simulink model "reactor_2"  (R2021a)
settings: Solver=VariableStepAuto  StartTime=0.0  StopTime=10.0  RelTol=1e-3
values from neighbouring files (symbols this model uses):
  c0 = 5.4698    [script.m]
  ci = 10    [script.m]
  EdR = 49584/8.32    (= 5959.61538462)    [script.m]
  hA = kT*At    (= 18821.555234)    [script.m]
  k0 = 34930800    [script.m]
  mdH = 24953    [script.m]
  q = 10    [script.m]
  rcp = 2093    [script.m]
  T0 = 339.437    [script.m]
  Ti = 38+273    (= 311)    [script.m]
  Tr = Tri    (= 311)    [script.m]
  V = 10    [script.m]
settings Model: Creator=Automatica  LastModifiedBy=Automatica

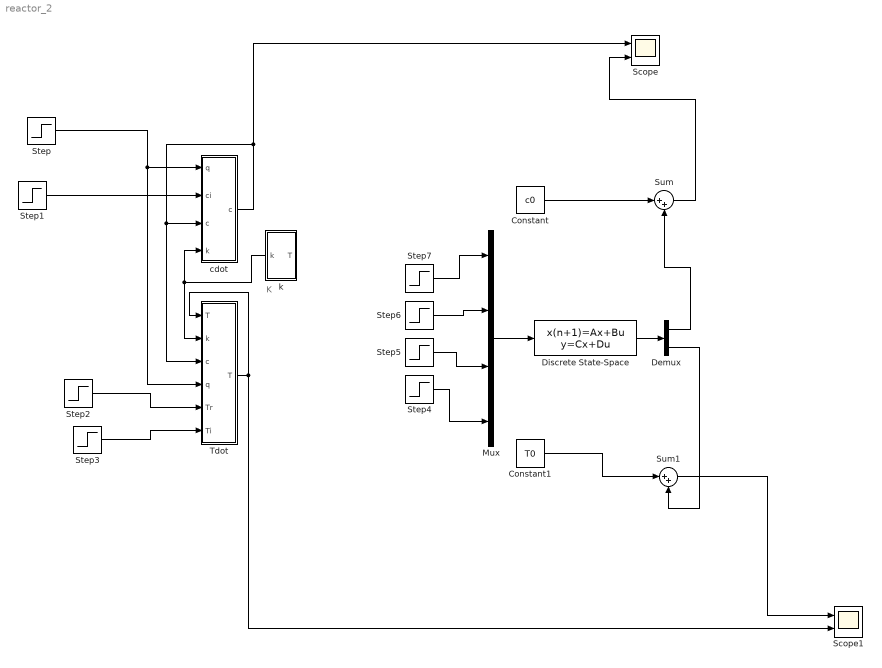
== system reactor_2 ==
  note: K
  Constant : Constant  Value=c0
  Constant1 : Constant  Value=T0
  Demux : Demux  Outputs=2
  Discrete State-Space : DiscreteStateSpace  SampleTime=-1
  Mux : Mux
  Scope : Scope  NumInputPorts=2
  Scope1 : Scope  NumInputPorts=2
  Step : Step  Time=0  Before=q  After=1.1*q  SampleTime=0
  Step1 : Step  Time=0  Before=ci  After=1.1*ci  SampleTime=0
  Step2 : Step  Time=0  Before=Tr  After=1.1*Tr  SampleTime=0
  Step3 : Step  Time=0  Before=Ti  After=1.1*Ti  SampleTime=0
  Step4 : Step  Time=0  After=0.1*Ti  SampleTime=0
  Step5 : Step  Time=0  After=0.1*Tr  SampleTime=0
  Step6 : Step  Time=0  After=0.1*ci  SampleTime=0
  Step7 : Step  Time=0  After=0.1*q  SampleTime=0
  Sum : Sum  Inputs=|++
  Sum1 : Sum  Inputs=|++
  Tdot : Subsystem
  cdot : Subsystem
  k : Subsystem
  wires:
  Step2/1 -> Tdot/5(Tr)
  Step1/1 -> cdot/2(ci)
  Step3/1 -> Tdot/6(Ti)
  Step/1 -> cdot/1(q), Tdot/4(q)
  Tdot/1("T  ") -> Scope1/2, Tdot/1(T)
  cdot/1(c) -> Scope/1, cdot/3("c  "), Tdot/3(c)
  Step7/1 -> Mux/1
  Step6/1 -> Mux/2
  Step5/1 -> Mux/3
  Step4/1 -> Mux/4
  Mux/1 -> Discrete State-Space/1
  Discrete State-Space/1 -> Demux/1
  Demux/1 -> Sum/2
  Constant/1 -> Sum/1
  Sum/1 -> Scope/2
  Constant1/1 -> Sum1/1
  Demux/2 -> Sum1/2
  Sum1/1 -> Scope1/1
  k/1(k) -> Tdot/2(k), cdot/4(k)

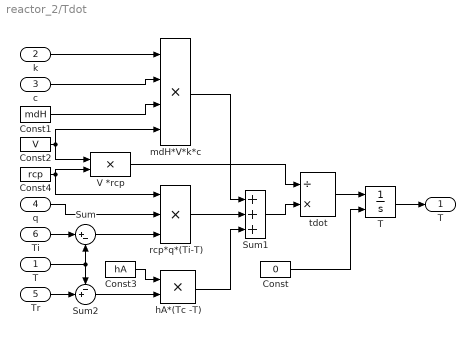
== system reactor_2/Tdot ==
  T : Inport  Interpolate=off
  k : Inport  Port=2  Interpolate=off
  c : Inport  Port=3  Interpolate=off
  q : Inport  Port=4  Interpolate=off
  Tr : Inport  Port=5  Interpolate=off
  Ti : Inport  Port=6  Interpolate=off
  Const : Constant  Value=0
  Const1 : Constant  Value=mdH
  Const2 : Constant  Value=V
  Const3 : Constant  Value=hA
  Const4 : Constant  Value=rcp
  Sum : Sum  Inputs=|+-  InputSameDT=on  SaturateOnIntegerOverflow=on  OutDataTypeStr=Inherit: Same as first input
  Sum1 : Sum  Inputs=+++  InputSameDT=on  SaturateOnIntegerOverflow=on  OutDataTypeStr=Inherit: Same as first input
  Sum2 : Sum  Inputs=-+|  InputSameDT=on  SaturateOnIntegerOverflow=on  OutDataTypeStr=Inherit: Same as first input
  "T " : Integrator  InitialConditionSource=external
  V *rcp : Product  Inputs=**  InputSameDT=on  RndMeth=Zero  SaturateOnIntegerOverflow=on  OutDataTypeStr=Inherit: Same as first input
  hA*(Tc -T) : Product  Inputs=**  InputSameDT=on  RndMeth=Zero  SaturateOnIntegerOverflow=on  OutDataTypeStr=Inherit: Same as first input
  mdH*V*k*c : Product  Inputs=****  InputSameDT=on  RndMeth=Zero  SaturateOnIntegerOverflow=on  OutDataTypeStr=Inherit: Same as first input
  rcp*q*(Ti-T) : Product  Inputs=***  InputSameDT=on  RndMeth=Zero  SaturateOnIntegerOverflow=on  OutDataTypeStr=Inherit: Same as first input
  tdot : Product  Inputs=/*  InputSameDT=on  RndMeth=Zero  SaturateOnIntegerOverflow=on  OutDataTypeStr=Inherit: Same as first input
  "T  " : Outport
  wires:
  Ti/1 -> Sum/1
  Sum/1 -> rcp*q*(Ti-T)/3
  q/1 -> rcp*q*(Ti-T)/2
  T/1 -> Sum/2, Sum2/1
  Tr/1 -> Sum2/2
  Sum2/1 -> hA*(Tc -T)/2
  Const3/1 -> hA*(Tc -T)/1
  k/1 -> mdH*V*k*c/1
  c/1 -> mdH*V*k*c/2
  Const1/1 -> mdH*V*k*c/3
  mdH*V*k*c/1 -> Sum1/1
  rcp*q*(Ti-T)/1 -> Sum1/2
  hA*(Tc -T)/1 -> Sum1/3
  Const2/1 -> mdH*V*k*c/4, V *rcp/1
  Const4/1 -> rcp*q*(Ti-T)/1, V *rcp/2
  V *rcp/1 -> tdot/1
  Sum1/1 -> tdot/2
  tdot/1 -> "T "/1
  Const/1 -> "T "/2
  "T "/1 -> "T  "/1

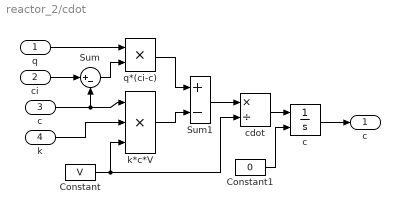
== system reactor_2/cdot ==
  q : Inport  Interpolate=off
  ci : Inport  Port=2  Interpolate=off
  "c  " : Inport  Port=3  Interpolate=off
  k : Inport  Port=4  Interpolate=off
  Constant : Constant  Value=V
  Constant1 : Constant  Value=0
  Sum : Sum  Inputs=|+-  InputSameDT=on  SaturateOnIntegerOverflow=on  OutDataTypeStr=Inherit: Same as first input
  Sum1 : Sum  Inputs=+-  InputSameDT=on  SaturateOnIntegerOverflow=on  OutDataTypeStr=Inherit: Same as first input
  "c " : Integrator  InitialConditionSource=external
  cdot : Product  Inputs=*/  InputSameDT=on  RndMeth=Zero  SaturateOnIntegerOverflow=on  OutDataTypeStr=Inherit: Same as first input
  k*c*V : Product  Inputs=***  InputSameDT=on  RndMeth=Zero  SaturateOnIntegerOverflow=on  OutDataTypeStr=Inherit: Same as first input
  q*(ci-c) : Product  Inputs=**  InputSameDT=on  RndMeth=Zero  SaturateOnIntegerOverflow=on  OutDataTypeStr=Inherit: Same as first input
  c : Outport
  wires:
  ci/1 -> Sum/1
  "c  "/1 -> k*c*V/1, Sum/2
  q/1 -> q*(ci-c)/1
  Sum/1 -> q*(ci-c)/2
  k/1 -> k*c*V/2
  q*(ci-c)/1 -> Sum1/1
  k*c*V/1 -> Sum1/2
  Sum1/1 -> cdot/1
  Constant/1 -> k*c*V/3, cdot/2
  cdot/1 -> "c "/1
  "c "/1 -> c/1
  Constant1/1 -> "c "/2

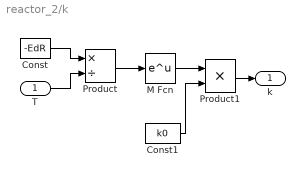
== system reactor_2/k ==
  T : Inport  Interpolate=off
  Const : Constant  Value=-EdR
  Const1 : Constant  Value=k0
  M Fcn : Math  SignedPower=on  SaturateOnIntegerOverflow=on
  Product : Product  Inputs=*/  InputSameDT=on  RndMeth=Zero  SaturateOnIntegerOverflow=on  OutDataTypeStr=Inherit: Same as first input
  Product1 : Product  Inputs=**  InputSameDT=on  RndMeth=Zero  SaturateOnIntegerOverflow=on  OutDataTypeStr=Inherit: Same as first input
  k : Outport
  wires:
  Const/1 -> Product/1
  T/1 -> Product/2
  Product/1 -> M Fcn/1
  M Fcn/1 -> Product1/1
  Const1/1 -> Product1/2
  Product1/1 -> k/1
